simulink model "model_main4"  (R2024b)
settings: Solver=ode4  StartTime=0.0  StopTime=1000  FixedStep=dt  RelTol=1e-3
undefined symbols (not defined in the file): dt, Iws, m_tot, norm_Ib, Omega1_init, Omega2_init, Omega3_init, Omega4_init, qb0, rad2rpm, RCS_F, RCS_F_vec, RCS_Pos, RCS_pos, RCS_PWM_Freq, RCS_Sampling_time, RCS_THR_vec, REL_TS_POS_I_0, REL_TS_VEL_I_0, rpm2rad, RW_As, RW_Max_Speed, RW_t_max, SC_Ib, SC_state0, SS_Total_Mass, TC_Kepler, TS_Ib, TS_qb0, TS_state0, TS_wb0, wb0
libraries: simulink x16, simulink_extras x15, aerolibutil x8, sharedtransform x8
(part 2 of 3)

== matlab function model_main4/Subsystem/Attitude_PD_control1 ==
  settings: updateMethod=DISCRETE
  data: F_B_cmd output; r_I input; v_I input; q_IB input; r_d input; v_d input; a_d input; m input
function F_B_cmd  = CTRL_WRENCH_6DOF(r_I, v_I, q_IB, r_d, v_d, a_d, m)
%#codegen
% ============================================================
% Controller block
% Input :
%   r_I      [3x1] current position in inertial frame
%   v_I      [3x1] current velocity in inertial frame
%   q_IB     [4x1] quaternion [qw qx qy qz], Body -> Inertial
%   omega_B  [3x1] current angular velocity in body frame
%
%   r_d      [3x1] desired position in inertial frame
%   v_d      [3x1] desired velocity in inertial frame
%   a_d      [3x1] desired acceleration in inertial frame
%   q_d      [4x1] desired quaternion, Body -> Inertial
%   omega_d_B[3x1] desired angular velocity in body frame
%
%   m        scalar mass
%   J        [3x3] inertia matrix in body frame
%
% Output:
%   F_B_cmd    [3x1] desired total body force
%   tau_B_cmd  [3x1] desired total body torque
% ============================================================

    % -------------------------
    % Quaternion normalize
    % -------------------------
    q_IB = quat_normalize(q_IB); 

    % -------------------------
    % Gains (example)
    % -------------------------
    Kp_r = 10*diag([0.01, 0.006, 0.006]);   % position gain
    Kd_r = 100*diag([0.01, 0.01, 0.01]);   % velocity damping
 
    % Kp_r = diag([0.010, 0.010, 0.010]);   % position gain
    % Kd_r = diag([0.060, 0.060, 0.060]);   % velocity damping

    % -------------------------
    % Position control
    % inertial acceleration command
    % -------------------------
    e_r = r_I - r_d;
    e_v = v_I - v_d;

    a_cmd   = a_d - Kp_r * e_r - Kd_r * e_v;
    F_I_cmd = m * a_cmd;

    % Convert inertial force -> body force
    R_IB    = quat_to_rotm(q_IB);
    F_B_cmd = R_IB.' * F_I_cmd;
 
end


% ============================================================
% Local helper functions
% ============================================================

function qn = quat_normalize(q)
    n = norm(q);
    if n < 1e-12
        qn = [1;0;0;0];
    else
        qn = q / n;
    end
end
 

function R = quat_to_rotm(q)
    % q = [qw qx qy qz], Body -> Inertial
    qw = q(1); qx = q(2); qy = q(3); qz = q(4);

    R = [1-2*(qy^2+qz^2),   2*(qx*qy-qz*qw),   2*(qx*qz+qy*qw);
         2*(qx*qy+qz*qw),   1-2*(qx^2+qz^2),   2*(qy*qz-qx*qw);
         2*(qx*qz-qy*qw),   2*(qy*qz+qx*qw),   1-2*(qx^2+qy^2)];
end

== matlab function model_main4/Subsystem/Thruster Allocation ==
  settings: updateMethod=DISCRETE
  data: u_pwm output; F_B_cmd input; tau_B_cmd input; F_B_real output; tau_B_real output; r input; d input; F_max input
function [u_pwm, F_B_real, tau_B_real] = ALLOC_THRUSTER_PWM_16(F_B_cmd, tau_B_cmd, r, d, F_max)
%#codegen
% ============================================================
% Allocation block
% Input :
%   F_B_cmd    [3x1] desired total body force
%   tau_B_cmd  [3x1] desired total body torque
%
% Output:
%   u_pwm      [12x1] thruster duty command, 0 ~ 1
%   F_B_real   [3x1] realized body force after allocation
%   tau_B_real [3x1] realized body torque after allocation
%
% Example:
%   12-thruster layout for 6DoF control
%   Replace thruster geometry / Tmax below with your real spacecraft values.
% ============================================================

    % Build 6x12 thruster mapping matrix A
    A = build_thruster_matrix( 16, r, d, F_max);

    % Desired wrench
    w_cmd = [F_B_cmd; tau_B_cmd];

    % Bounded least-squares allocation: 0 <= u <= 1
    u_pwm = bounded_allocator_0_1(A, w_cmd);

    % Realized wrench
    w_real     = A * u_pwm;
    F_B_real   = w_real(1:3);
    tau_B_real = w_real(4:6);
end


% ============================================================
% Thruster layout
% ============================================================
function A = build_thruster_matrix(N, r, d, F_max)
    % --------------------------------------------------------
    % Example spacecraft half-size [m]
    % Replace with your real geometry
    % --------------------------------------------------------
    % L = 0.50;   % lever arm

    % --------------------------------------------------------
    % Max thrust of each thruster [N]
    % Replace with your real thruster max force
    % --------------------------------------------------------
    Tmax = F_max * ones(N,1);

    % --------------------------------------------------------
    % Thruster positions r_i in body frame [m]
    % Each column is one thruster position
    % --------------------------------------------------------
    % r = [ ...
    %      0,   0,   0,   0,   L,  -L,   L,  -L,   L,  -L,   L,  -L;
    %      L,  -L,   L,  -L,   0,   0,   0,   0,   L,   L,  -L,  -L;
    %      L,  -L,  -L,   L,   L,  -L,  -L,   L,   0,   0,   0,   0 ];

    % --------------------------------------------------------
    % Thruster unit directions d_i in body frame
    %
    % T1,T2 : +X
    % T3,T4 : -X
    % T5,T6 : +Y
    % T7,T8 : -Y
    % T9,T10: +Z
    % T11,T12:-Z
    % --------------------------------------------------------
    % d = [ ...
    %      1,   1,  -1,  -1,   0,   0,   0,   0,   0,   0,   0,   0;
    %      0,   0,   0,   0,   1,   1,  -1,  -1,   0,   0,   0,   0;
    %      0,   0,   0,   0,   0,   0,   0,   0,   1,   1,  -1,  -1 ];

    % --------------------------------------------------------
    % Build A = [F; tau], size 6x12
    % --------------------------------------------------------
    A = zeros(6,N);

    for i = 1:N
        f_i       = Tmax(i) * d(:,i);
        tau_i     = cross(r(:,i), f_i);
        A(:,i)    = [f_i; tau_i];
    end
end


% ============================================================
% Bounded allocator: 0 <= u <= 1
% Codegen-friendly fixed-size active-set style
% ============================================================
function u = bounded_allocator_0_1(A, w_cmd)
    N = 16;
    u = zeros(N,1);

    % free_mask(i)=true means this thruster is still free to solve
    free_mask = true(N,1);

    lambda = 1e-8;   % small damping

    for iter = 1:(N+1)

        % Residual after fixed/saturated thrusters
        w_res = w_cmd;
        for i = 1:N
            if ~free_mask(i)
                w_res = w_res - A(:,i) * u(i);
            end
        end

        % Collect free columns into Af (fixed-size construction)
        Af  = zeros(6,N);
        idx = zeros(N,1);
        nf  = 0;

        for i = 1:N
            if free_mask(i)
                nf = nf + 1;
                idx(nf) = i;
                Af(:,nf) = A(:,i);
            end
        end

        if nf == 0
            break;
        end

        % Minimum-norm damped solution on free set
        M       = Af * Af.' + lambda * eye(6);
        uf_full = Af.' * (M \ w_res);   % size Nx1, only first nf entries used

        % Put candidate solution into u
        for k = 1:nf
            i = idx(k);
            u(i) = uf_full(k);
        end

        % Check bounds and fix saturated variables
        violated = false;
        for k = 1:nf
            i = idx(k);

            if u(i) < 0
                u(i) = 0;
                free_mask(i) = false;
                violated = true;

            elseif u(i) > 1
                u(i) = 1;
                free_mask(i) = false;
                violated = true;
            end
        end

        if ~violated
            break;
        end
    end

    % Final clipping
    for i = 1:N
        if u(i) < 0
            u(i) = 0;
        elseif u(i) > 1
            u(i) = 1;
        end
    end
end

== matlab function model_main4/saturation ==
  data: max_speed input; res output; Omega_mea input; torque_cmd input
function res  = saturation(max_speed, Omega_mea, torque_cmd)

Omega1_mea = Omega_mea(1);
Omega2_mea = Omega_mea(2);
Omega3_mea = Omega_mea(3);
Omega4_mea = Omega_mea(4);

if abs(Omega1_mea)> max_speed
    res1 = 0;
else
    res1 = torque_cmd(1);
end

if abs(Omega2_mea)>max_speed
    res2 = 0;
else
    res2 = torque_cmd(2);
end

if abs(Omega3_mea)>max_speed
    res3 = 0;
else
    res3 = torque_cmd(3);
end

if abs(Omega4_mea)>max_speed
    res4 = 0;
else
    res4 = torque_cmd(4);
end

res = [res1,res2,res3,res4]';

end

== matlab function model_main4/TS 6-DOF Dynamics ==
  data: w input; x input; Ib input; wd output; T_ext input; F_ext input; xd output
function [wd, xd]  = eq_propagate(w, x, Ib, T_ext, F_ext)
% % 
% 출력 1: 위성 동체 좌표계 각가속도
% 출력 2: 관성좌표계 선가속도

%% Rotational Motion
% wd = [0 0 0]';
wd = inv(Ib)*(T_ext - cross(w, Ib*w));

%% Translational Motion


u  = 3.9860064e+14; % earth gravitional parameter
Re = 6378137;      % earth radius [m]

xd = zeros(size(x));

v1_i = x(4); % x1 = dx/dt
v2_i = x(5); % y1 = dy/dt
v3_i = x(6); % z1 = dz/dt
p1_i = x(1); % x
p2_i = x(2); % y
p3_i = x(3); % z

r=sqrt(p1_i^2+p2_i^2+p3_i^2);

% % %   Keplar Motion Equatnion
% % %  => r_dd + u/(r^3)r_ = 0 => r_dd = -u/(r^3)r_
xd(1) = v1_i;
xd(2) = v2_i;
xd(3) = v3_i;
xd(4) = -u*p1_i/(r^3) +  F_ext(1);
xd(5) = -u*p2_i/(r^3) +  F_ext(2);
xd(6) = -u*p3_i/(r^3) +  F_ext(3);

end

== matlab function model_main4/Subsystem/Attitude_PD_control2 ==
  settings: updateMethod=DISCRETE
  data: q_err input; omega_B input; omega_d_B input; J input; tau_B_cmd output
function tau_B_cmd  = CTRL_WRENCH_6DOF(q_err, omega_B, omega_d_B, J)
%#codegen
% ============================================================
% Controller block
% Input :
%   r_I      [3x1] current position in inertial frame
%   v_I      [3x1] current velocity in inertial frame
%   q_IB     [4x1] quaternion [qw qx qy qz], Body -> Inertial
%   omega_B  [3x1] current angular velocity in body frame
%
%   r_d      [3x1] desired position in inertial frame
%   v_d      [3x1] desired velocity in inertial frame
%   a_d      [3x1] desired acceleration in inertial frame
%   q_d      [4x1] desired quaternion, Body -> Inertial
%   omega_d_B[3x1] desired angular velocity in body frame
%
%   m        scalar mass
%   J        [3x3] inertia matrix in body frame
%
% Output:
%   F_B_cmd    [3x1] desired total body force
%   tau_B_cmd  [3x1] desired total body torque
% ============================================================
 
    % -------------------------
    % Gains (example)
    % -------------------------
    Kq   = J*diag([0.3, 0.3, 0.3]);   % attitude gain
    Kw   = J*diag([5, 5, 5]);   % angular-rate damping

    % Kq   = diag([10.0, 10.0, 10.0]);   % attitude gain
    % Kw   = diag([6.0,  6.0,  6.0 ]);   % angular-rate damping
    % -------------------------
 
    % -------------------------
    % Attitude control 
    % -------------------------
 
    % shortest-path quaternion
    if q_err(1) < 0
        q_err = -q_err;
    end

    e_w = omega_B - omega_d_B;

    % PD + gyro compensation
    tau_B_cmd = -Kq * q_err(2:4) ...
                -Kw * e_w ...
                +cross(omega_B, J * omega_B);
end


% ============================================================
% Local helper functions
% ============================================================

function qn = quat_normalize(q)
    n = norm(q);
    if n < 1e-12
        qn = [1;0;0;0];
    else
        qn = q / n;
    end
end

function qc = quat_conj(q)
    qc = [q(1); -q(2); -q(3); -q(4)];
end

function q = quat_mul(q1, q2)
    % Hamilton product
    w1 = q1(1); x1 = q1(2); y1 = q1(3); z1 = q1(4);
    w2 = q2(1); x2 = q2(2); y2 = q2(3); z2 = q2(4);

    q = [ w1*w2 - x1*x2 - y1*y2 - z1*z2;
          w1*x2 + x1*w2 + y1*z2 - z1*y2;
          w1*y2 - x1*z2 + y1*w2 + z1*x2;
          w1*z2 + x1*y2 - y1*x2 + z1*w2 ];
end

== matlab function model_main4/RCS_Position&Attitude_Controller ==
  settings: updateMethod=DISCRETE
  data: r_rel input; v_rel input; r_ref input; v_ref input; a_ref input; q input; q_err input; w_err input; wb input; F_cmd_B output; tau_cmd_B output; m_sc input; Ib input; Kp_pos input; Kd_pos input; Kp_att input; Kd_att input; r_err output; v_err output; q output; q_err_vec output; w_err output; a_cmd output
function [F_cmd_B, tau_cmd_B, r_err, v_err, q, q_err_vec, w_err, a_cmd] = ...
    relative_position_los_controller( ...
    r_rel, v_rel, ...          % [3x1] relative position/velocity
    r_ref, v_ref, a_ref, ...   % [3x1] desired relative pos/vel/acc
    q, q_err, w_err, wb, m_sc, Ib, Kp_pos, Kd_pos, Kp_att, Kd_att)
%#codegen
%
% q, q_los_ref : scalar-first quaternion [qw qx qy qz]'
%                body -> reference
% r_rel, r_ref, v_rel, v_ref, a_ref : reference frame 기준
%
% 출력:
% F_cmd_B   : [3x1] body frame force command
% tau_cmd_B : [3x1] body frame torque command

F_cmd_B   = zeros(3,1);
tau_cmd_B = zeros(3,1);
r_err     = zeros(3,1);
v_err     = zeros(3,1);
q_err_vec = zeros(3,1);
% w_err     = zeros(3,1);
a_cmd     = zeros(3,1);

%% 1) Relative position controller
r_err = r_ref - r_rel;
v_err = v_ref - v_rel;

a_cmd = a_ref + Kp_pos * r_err + Kd_pos * v_err;
F_cmd_R = m_sc * a_cmd;

%% 2) Reference frame -> body frame
% q : body -> reference
% therefore F_B = C_BR' * F_R
C_BR   = quat_to_dcm_sf(q);
F_cmd_B = C_BR' * F_cmd_R;

%% 3) LOS attitude controller

% shortest path
% if q_err(1) < 0
%     q_err = -q_err;
% end

q_err_vec = q_err(2:4);

tau_cmd_B = Kp_att * q_err_vec + Kd_att * w_err + cross(wb, Ib*wb);
end


function q_out = quat_mul_sf(a, b)
% scalar-first quaternion multiplication
q_out = [ a(1)*b(1) - a(2)*b(2) - a(3)*b(3) - a(4)*b(4);
    a(1)*b(2) + a(2)*b(1) + a(3)*b(4) - a(4)*b(3);
    a(1)*b(3) - a(2)*b(4) + a(3)*b(1) + a(4)*b(2);
    a(1)*b(4) + a(2)*b(3) - a(3)*b(2) + a(4)*b(1) ];
end


function C = quat_to_dcm_sf(q)
% scalar-first quaternion, body -> reference
q = q / (sqrt(sum(q.^2)) + 1e-12);

qw = q(1);
qx = q(2);
qy = q(3);
qz = q(4);

C = [1-2*(qy*qy+qz*qz),   2*(qx*qy-qw*qz),   2*(qx*qz+qw*qy);
    2*(qx*qy+qw*qz),     1-2*(qx*qx+qz*qz), 2*(qy*qz-qw*qx);
    2*(qx*qz-qw*qy),     2*(qy*qz+qw*qx),   1-2*(qx*qx+qy*qy)];
end

== matlab function model_main4/RCS_Force_Torque_Allocation ==
  settings: updateMethod=DISCRETE
  data: F_cmd input; tau_cmd input; RCS_pos input; RCS_F_vec input; Tmax input; duty output; F_est output; tau_est output; F_err output; tau_err output; sat_ratio output; wF input; wT input
function [duty, F_est, tau_est, F_err, tau_err, sat_ratio] = ...
    rcs_force_torque_allocator(F_cmd, tau_cmd, RCS_pos, RCS_F_vec, Tmax, wF, wT)
%#codegen
%
% F_cmd      : [3x1] commanded force in body frame [N]
% tau_cmd    : [3x1] commanded torque in body frame [N*m]
% RCS_pos    : [3xN] thruster positions in body frame [m]
% RCS_F_vec  : [3xN] thruster direction vectors
% Tmax       : scalar, max thrust of one thruster [N]
% wF         : scalar, force tracking weight
% wT         : scalar, torque tracking weight
%
% duty       : [N x 1], 0~1
% F_est      : [3x1], achieved force [N]
% tau_est    : [3x1], achieved torque [N*m]
% F_err      : [3x1], force error [N]
% tau_err    : [3x1], torque error [N*m]
% sat_ratio  : saturated thruster ratio

    N = size(RCS_pos, 2);

    duty      = zeros(N,1);
    F_est     = zeros(3,1);
    tau_est   = zeros(3,1);
    F_err     = zeros(3,1);
    tau_err   = zeros(3,1);
    sat_ratio = 0;

    Fmat = zeros(3, N);
    Tmat = zeros(3, N);

    for i = 1:N
        dir_i = RCS_F_vec(:,i);
        nrm   = sqrt(sum(dir_i.^2));

        if nrm > 1e-12
            dir_i = dir_i / nrm;
        else
            dir_i = [0;0;0];
        end

        Fi = Tmax * dir_i;
        Ti = cross3(RCS_pos(:,i), Fi);

        Fmat(:,i) = Fi;
        Tmat(:,i) = Ti;
    end

    % Solve:
    % min || wF*(Fmat*u - F_cmd) ||^2 + || wT*(Tmat*u - tau_cmd) ||^2
    % s.t. 0 <= u <= 1

    A = [wF * Fmat;
         wT * Tmat];

    b = [wF * F_cmd;
         wT * tau_cmd];

    H = A' * A + 1e-8 * eye(N);
    g = A' * b;

    alpha = 1.0 / (trace(H) + 1e-9);
    u = zeros(N,1);

    for k = 1:150
        grad = H * u - g;
        u    = u - alpha * grad;

        for j = 1:N
            if u(j) < 0
                u(j) = 0;
            elseif u(j) > 1
                u(j) = 1;
            end
        end
    end

    duty    = u;
    F_est   = Fmat * duty;
    tau_est = Tmat * duty;

    F_err   = F_cmd   - F_est;
    tau_err = tau_cmd - tau_est;

    sat_ratio = sum(duty > 0.999) / N;
end


function c = cross3(a, b)
    c = [ a(2)*b(3) - a(3)*b(2);
          a(3)*b(1) - a(1)*b(3);
          a(1)*b(2) - a(2)*b(1) ];
end

== matlab function model_main4/Mission_Supporter ==
  settings: updateMethod=DISCRETE
  data: flag output; res_pos input; stop output; Los_angle input
function [flag, stop]  = Mission_Supporter(res_pos, Los_angle)
persistent prev_flag

if isempty(prev_flag)
    prev_flag = 0;
end

d_norm = norm(res_pos);
d_parking = 5;


if d_norm - d_parking > 1 
    prev_flag = 0; % approach, RCS on
else
    if prev_flag == 0 && Los_angle < 0.2
        prev_flag = 1; % station keeping, RW on
    end
end
 
flag= prev_flag;
 

% 종료 조건
if d_norm <= 0.1
    stop = 1;
else
    stop = 0;
end

== matlab function model_main4/command_generator ==
  settings: updateMethod=DISCRETE
  data: rel_p_cmd output; flag input; rel_v_cmd output; Kp_pos output; Kd_pos output
function [rel_p_cmd,rel_v_cmd,Kp_pos,Kd_pos]  = Mission_Supporter(flag)

if flag == 0
    rel_p_cmd = [5 0 0]';
    rel_v_cmd = [0 0 0]';
    Kp_pos = 0.3;
    Kd_pos = 18.0;
else
    rel_p_cmd = [1 0 0]';
    rel_v_cmd = [0 0 0]';
    Kp_pos = 0.3;
    Kd_pos = 18.0;    
end


end

== matlab function model_main4/Get LOS Quaternion ==
  data: r_rel input; q output; ang_deg output; axis_rot output
function [q, ang_deg, axis_rot] = boresight_to_target_quat(r_rel)
%#codegen
% ============================================================
% boresight_to_target_quat
%
% Input:
%   r_rel    [3x1] : relative position vector
%
% Output:
%   q        [4x1] : quaternion [w; x; y; z]
%                    rotating boresight [1;0;0] to r_rel direction
%   ang_deg  [1x1] : rotation angle in degrees
%   axis_rot [3x1] : rotation axis (unit vector)
%
% Notes:
%   - boresight reference is fixed as [1; 0; 0]
%   - quaternion is scalar-first
%   - handles parallel / anti-parallel edge cases
% ============================================================

    % Reference boresight
    b_ref = [1; 0; 0];

    % Small threshold
    eps_val = 1e-12;

    % Check input norm
    r_norm = norm(r_rel);
    if r_norm < eps_val
        % Undefined direction
        q = [1; 0; 0; 0];
        ang_deg = 0;
        axis_rot = [1; 0; 0];
        return;
    end

    % Normalize target direction
    v = r_rel / r_norm;
    u = b_ref;

    % Dot product
    c = dot(u, v);
    c = max(min(c, 1.0), -1.0);   % numerical safety

    % Case 1: same direction
    if c > 1 - 1e-10
        q = [1; 0; 0; 0];
        ang_deg = 0;
        axis_rot = [1; 0; 0];
        return;
    end

    % Case 2: opposite direction
    if c < -1 + 1e-10
        % Need 180 deg rotation about any axis orthogonal to [1;0;0]
        % Choose y-axis
        axis_rot = [0; 1; 0];
        q = [0; axis_rot];   % cos(pi/2)=0, sin(pi/2)=1
        ang_deg = 180;
        return;
    end

    % General case
    cross_uv = cross(u, v);

    % Robust quaternion from two vectors:
    % q = [1 + dot(u,v); cross(u,v)] then normalize
    q = [1 + c;
         cross_uv(1);
         cross_uv(2);
         cross_uv(3)];

    q = q / norm(q);

    % Rotation angle
    ang_rad = 2 * acos(q(1));
    ang_deg = ang_rad * 180 / pi;

    % Rotation axis
    s = sqrt(1 - q(1)^2);
    if s < 1e-10
        axis_rot = [1; 0; 0];
    else
        axis_rot = q(2:4) / s;
    end
end

== matlab function model_main4/Enabled Subsystem/QP Controller ==
  settings: updateMethod=DISCRETE
  data: tau_pd input; u_rw_cmd output; Omega_rw input; RW_max_speed input; tau_rcs_max input; eta_rcs input; v1 input; v2 input; dt input; tau_rcs_cmd output; tau_rw_body output; tau_dump_ref output; s1 output; s2 output; exitflag_out output
function [u_rw_cmd, tau_rcs_cmd, tau_rw_body, tau_dump_ref, s1, s2, exitflag_out] = ...
    QP_Controller(tau_pd, Omega_rw, RW_max_speed, tau_rcs_max, eta_rcs, v1, v2, dt)
 
% QP with two slack variables:
%   s1 : attitude torque slack
%   s2 : dumping torque slack
%
% Inputs
%   tau_pd       [3x1] desired total body torque from PD [N*m]
%   Omega_rw     [4x1] current wheel speeds [rad/s]
%   RW_max_speed [1x1] wheel speed limit [rad/s]
%   tau_rcs_max  [3x1] approximate RCS body torque bound [N*m]
%   eta_rcs      [1x1] RCS effort weight
%   v1           [1x1] attitude slack weight
%   v2           [1x1] dumping slack weight
%   dt           [1x1] sample time [s]
%
% Outputs
%   u_rw_cmd     [4x1] RW wheel torque command [N*m]
%   tau_rcs_cmd  [3x1] RCS dumping body torque command [N*m]
%   tau_rw_body  [3x1] RW body torque [N*m]
%   tau_dump_ref [3x1] desired dumping torque reference [N*m]
%   s1           [3x1] attitude torque slack [N*m]
%   s2           [3x1] dumping torque slack [N*m]
%   exitflag_out [1x1] quadprog exitflag

persistent u_save;

if isempty(u_save)
    u_save = zeros(13,1);
end
 
u_prev   = u_save;

tau_pd      = reshape(tau_pd,      [3,1]);
Omega_rw    = reshape(Omega_rw,    [4,1]);
tau_rcs_max = reshape(tau_rcs_max, [3,1]);
Omega_ref = 1000 * pi/30 * ones(4,1);

%% RW geometry from current model
% tau_rw_body = -As * u_rw_cmd
As = [ 0.70710678,  0.0,        -0.70710678,  0.0;
       0.0,         0.70710678,  0.0,        -0.70710678;
       0.70710678,  0.70710678,  0.70710678,  0.70710678 ];

Iws = 0.227 * eye(4);

%% wheel limits
% Wheel torque limits [N*m]
u_rw_max = 0.5 * ones(4,1);
u_rw_min = -u_rw_max;

% Wheel torque rate limits [N*m/s]
du_max = [0.50; 0.50; 0.50; 0.50]*100;
du_min = -du_max;

% Wheel speed limits [rad/s]
Omega_max = RW_max_speed * ones(4,1);
Omega_min = -Omega_max;

%% dumping reference
% % saturation ratio
% sat_ratio = max(abs(Omega_rw) ./ (Omega_max + 1e-12));
% 
% % activation factor alpha
% if sat_ratio <= sat_start
%     alpha = 0.0;
% else
%     alpha = (sat_ratio - sat_start) / (1.0 - sat_start);
%     if alpha > 1.0
%         alpha = 1.0;
%     end
% end
alpha =  0;
tau_dump_ref = -alpha * As * Iws * (Omega_rw - Omega_ref);

% % approximate RCS torque clipping
% for i = 1:3
%     if tau_dump_ref(i) > tau_rcs_max(i)
%         tau_dump_ref(i) = tau_rcs_max(i);
%     elseif tau_dump_ref(i) < -tau_rcs_max(i)
%         tau_dump_ref(i) = -tau_rcs_max(i);
%     end
% end

%% decision variable
% z = [u_rw(4); tau_rcs(3); s1(3); s2(3)]  => total 13

%% cost

Wu   = eye(4);
Wrcs = eta_rcs * eye(3);
V1   = v1      * eye(3);
V2   = v2      * eye(3);

H = blkdiag(Wu, Wrcs, V1, V2);
H = 0.5*(H + H') + 1e-9*eye(13);

f = zeros(13,1);

%% equality constraints
% 1) attitude torque:
%    -As*u_rw + tau_rcs - s1 = tau_pd
%
% 2) dumping torque:
%    tau_rcs - s2 = tau_dump_ref

Aeq = [       -As, eye(3),     -eye(3), zeros(3,3);
       zeros(3,4), eye(3),  zeros(3,3),    -eye(3)];

beq = [      tau_pd;
       tau_dump_ref];

%% bounds
% RW torque bounds
% Torque-rate bounds
lb_rate = u_prev(1:4) + du_min * dt;
ub_rate = u_prev(1:4) + du_max * dt;

% Speed-next bounds
% Omega_next = Omega_rw + dt*(u./Jw)
% => u >= Jw .* (Omega_min - Omega_rw)/dt
% => u <= Jw .* (Omega_max - Omega_rw)/dt
lb_speed = diag(Iws) .* ((Omega_min - Omega_rw) / dt);
ub_speed = diag(Iws) .* ((Omega_max - Omega_rw) / dt);

% Final bounds
lb_u = inf*max(u_rw_min, max(lb_rate, lb_speed));
ub_u = min(u_rw_max, min(ub_rate, ub_speed));

% Feasibility repair
% for i = 1:4
%     if lb_u(i) > ub_u(i)
%         c = 0.5 * (lb_u(i) + ub_u(i));
%         lb_u(i) = c;
%         ub_u(i) = c;
%     end
% end


% RCS torque bounds
% lb_t = -tau_rcs_max;
% ub_t =  tau_rcs_max;
lb_t = -inf*ones(3,1);
ub_t =  inf*ones(3,1);

% slack bounds
big = 1e6;  % inf
lb_s1 = -big * ones(3,1);
ub_s1 =  big * ones(3,1);
lb_s2 = -big * ones(3,1);
ub_s2 =  big * ones(3,1);

lb = [lb_u; lb_t; lb_s1; lb_s2];
ub = [ub_u; ub_t; ub_s1; ub_s2];

%% initial guess
x0 = [zeros(4,1);
      zeros(3,1);
      -tau_pd;
      -tau_dump_ref];
% rw : Omegad cmd, rcs : tau cmd, 
% x0 = min(max(u_prev, lb), ub);

%% solve
options = optimoptions('quadprog', ...
    'Algorithm', 'active-set', ...
    'Display', 'off', ...
    'ConstraintTolerance', 1e-6, ...
    'OptimalityTolerance', 1e-6, ...
    'StepTolerance', 1e-12, ...
    'MaxIterations', 50);

[z, ~, exitflag] = quadprog(H, f, [], [], Aeq, beq, lb, ub, x0, options);

if isempty(z) || exitflag <= 0
    z = x0;
end

%% outputs
u_rw_cmd    = z(1:4);
tau_rcs_cmd = z(5:7);
s1          = z(8:10);
s2          = z(11:13);

tau_rw_body = -As * u_rw_cmd;
% tau_total   = tau_rw_body + tau_rcs_cmd;
u_save = z;
exitflag_out = exitflag;
end

== matlab function model_main4/Enabled Subsystem/QP Controller1 ==
  settings: updateMethod=DISCRETE
  data: tau_pd_in input; u_rw_cmd output; Omega_rw_in input; Omega_ref_in input; RW_max_speed input; tau_rcs_max_in input; k_dump input; eta_rw input; eta_rcs input; v1 input; v2 input; dt input; tau_rcs_cmd output; tau_rw_body output; tau_dump_ref output; s1 output; s2 output; exitflag_out output
function [u_rw_cmd, tau_rcs_cmd, tau_rw_body, tau_dump_ref, s1, s2, exitflag_out] = ...
    QP_CA_RW_RCS3(tau_pd_in, Omega_rw_in, Omega_ref_in, ...
                  RW_max_speed, tau_rcs_max_in, ...
                  k_dump, eta_rw, eta_rcs, v1, v2, dt)
%#codegen
%
% QP control allocation based on the structure of Sec. 3.1,
% simplified to:
%   - RW (internal actuator)
%   - lumped 3-axis external torque command (for later RCS allocation)
%
% Decision variable:
%   z = [u_rw(4); tau_rcs(3); s1(3); s2(3)]  -> 13 states
%
% Equality constraints:
%   -As*u_rw + tau_rcs - s1 = tau_pd
%    tau_rcs - s2           = tau_dump_ref
%
% Inputs
%   tau_pd_in      [3x1] desired attitude body torque from high-level controller [N*m]
%   Omega_rw_in    [4x1] current RW speeds [rad/s]
%   Omega_ref_in   [4x1] desired RW speed reference [rad/s]
%   RW_max_speed   [1x1] RW speed limit [rad/s]
%   tau_rcs_max_in [3x1] max body torque envelope available from RCS [N*m]
%   k_dump         [1x1] momentum dumping gain [1/s]
%   eta_rw         [1x1] RW effort weight
%   eta_rcs        [1x1] external torque effort weight
%   v1             [1x1] attitude slack weight
%   v2             [1x1] dumping slack weight
%   dt             [1x1] sample time [s]
%
% Outputs
%   u_rw_cmd       [4x1] RW motor torque command [N*m]
%   tau_rcs_cmd    [3x1] desired 3-axis body torque for RCS allocation [N*m]
%   tau_rw_body    [3x1] body torque generated by RW [N*m]
%   tau_dump_ref   [3x1] desired external dumping torque [N*m]
%   s1             [3x1] attitude torque slack
%   s2             [3x1] dumping torque slack
%   exitflag_out   [1x1] quadprog exitflag

persistent z_save;

if isempty(z_save)
    z_save = zeros(13,1);
end

%% outputs
u_rw_cmd     = zeros(4,1);
tau_rcs_cmd  = zeros(3,1);
tau_rw_body  = zeros(3,1);
tau_dump_ref = zeros(3,1);
s1           = zeros(3,1);
s2           = zeros(3,1);
exitflag_out = 0;

%% fixed-size local copies
tau_pd = zeros(3,1);
tau_pd(1) = tau_pd_in(1);
tau_pd(2) = tau_pd_in(2);
tau_pd(3) = tau_pd_in(3);

Omega_rw = zeros(4,1);
Omega_rw(1) = Omega_rw_in(1);
Omega_rw(2) = Omega_rw_in(2);
Omega_rw(3) = Omega_rw_in(3);
Omega_rw(4) = Omega_rw_in(4);

Omega_ref = zeros(4,1);
Omega_ref(1) = Omega_ref_in(1);
Omega_ref(2) = Omega_ref_in(2);
Omega_ref(3) = Omega_ref_in(3);
Omega_ref(4) = Omega_ref_in(4);

tau_rcs_max = zeros(3,1);
tau_rcs_max(1) = abs(tau_rcs_max_in(1));
tau_rcs_max(2) = abs(tau_rcs_max_in(2));
tau_rcs_max(3) = abs(tau_rcs_max_in(3));

if dt <= 1e-6
    dt = 1e-6;
end

if RW_max_speed <= 1e-6
    RW_max_speed = 1e-6;
end

%% RW geometry
% tau_rw_body = -As * u_rw
As = [ 0.70710678,  0.0,        -0.70710678,  0.0;
       0.0,         0.70710678,  0.0,        -0.70710678;
       0.70710678,  0.70710678,  0.70710678,  0.70710678 ];

% wheel spin inertias [kg*m^2]
Jw = 0.227 * ones(4,1);

%% actuator limits
% RW torque limits
u_rw_max = 0.2 * ones(4,1);
u_rw_min = -u_rw_max;

% RW torque-rate limits
du_max = 2.0 * ones(4,1);   % [N*m/s]
du_min = -du_max;

% RW speed limits
Omega_max = RW_max_speed * ones(4,1);
Omega_min = -Omega_max;

%% previous solution
z_prev = z_save;
u_prev = z_prev(1:4);

%% virtual momentum dumping torque
% Paper uses u_h = -k_h * (...) * Cw*Jw*omega_w,e
% Here simplified for RCS-only external torque:
%   tau_dump_ref = -k_dump * h_rw_err
% where h_rw_err = As * diag(Jw) * (Omega_rw - Omega_ref)

omega_err = Omega_rw - Omega_ref;
h_rw_err  = As * (Jw .* omega_err);   % [N*m*s]
tau_dump_ref = -k_dump * h_rw_err;    % [N*m]

%% QP cost
% z = [u_rw(4); tau_rcs(3); s1(3); s2(3)]
H = zeros(13,13);
f = zeros(13,1);

% effort weights
H(1,1) = 2*eta_rw; H(2,2) = 2*eta_rw; H(3,3) = 2*eta_rw; H(4,4) = 2*eta_rw;
H(5,5) = 2*eta_rcs; H(6,6) = 2*eta_rcs; H(7,7) = 2*eta_rcs;
H(8,8) = 2*v1; H(9,9) = 2*v1; H(10,10) = 2*v1;
H(11,11) = 2*v2; H(12,12) = 2*v2; H(13,13) = 2*v2;

% optional small RW smoothing
wr = 1e-3;
H(1,1) = H(1,1) + 2*wr;
H(2,2) = H(2,2) + 2*wr;
H(3,3) = H(3,3) + 2*wr;
H(4,4) = H(4,4) + 2*wr;

f(1:4) = -2*wr*u_prev;

% numerical symmetry
H = 0.5*(H + H') + 1e-9*eye(13);

%% equality constraints
% -As*u_rw + tau_rcs - s1 = tau_pd
%  tau_rcs - s2           = tau_dump_ref

Aeq = [      -As, eye(3),    -eye(3), zeros(3,3);
       zeros(3,4), eye(3), zeros(3,3),   -eye(3)];

beq = [tau_pd;
       tau_dump_ref];

%% bounds
% RW torque-rate bounds
lb_rate = u_prev + du_min * dt;
ub_rate = u_prev + du_max * dt;

% RW speed-next bounds
% Omega_next = Omega_rw + dt*(u_rw./Jw)
lb_speed = Jw .* ((Omega_min - Omega_rw) / dt);
ub_speed = Jw .* ((Omega_max - Omega_rw) / dt);

% final RW bounds
lb_u = max(u_rw_min, max(lb_rate, lb_speed));
ub_u = min(u_rw_max, min(ub_rate, ub_speed));

% feasibility repair
for i = 1:4
    if lb_u(i) > ub_u(i)
        c = 0.5 * (lb_u(i) + ub_u(i));
        lb_u(i) = c;
        ub_u(i) = c;
    end
end

% external torque bounds
lb_t = -tau_rcs_max;
ub_t =  tau_rcs_max;

% slack bounds
big = 1e6;
lb_s1 = -big * ones(3,1);
ub_s1 =  big * ones(3,1);
lb_s2 = -big * ones(3,1);
ub_s2 =  big * ones(3,1);

lb = [lb_u; lb_t; lb_s1; lb_s2];
ub = [ub_u; ub_t; ub_s1; ub_s2];

%% initial guess (make it equality-feasible)
u0 = min(max(u_prev, lb_u), ub_u);

t0 = tau_dump_ref;
for i = 1:3
    if t0(i) > ub_t(i)
        t0(i) = ub_t(i);
    elseif t0(i) < lb_t(i)
        t0(i) = lb_t(i);
    end
end

s10 = -As*u0 + t0 - tau_pd;
s20 = t0 - tau_dump_ref;

x0 = [u0;
      t0;
      s10;
      s20];

%% solve
A = zeros(0,13);
b = zeros(0,1);

options = optimoptions('quadprog', ...
    'Algorithm', 'active-set', ...
    'Display', 'off', ...
    'ConstraintTolerance', 1e-6, ...
    'OptimalityTolerance', 1e-6, ...
    'StepTolerance', 1e-12, ...
    'MaxIterations', 50);

[z, ~, exitflag] = quadprog(H, f, A, b, Aeq, beq, lb, ub, x0, options);

if isempty(z) || exitflag <= 0
    z = x0;
end

%% outputs
u_rw_cmd    = z(1:4);
tau_rcs_cmd = z(5:7);
s1          = z(8:10);
s2          = z(11:13);

tau_rw_body = -As * u_rw_cmd;

z_save = z;
exitflag_out = exitflag;

end

== matlab function model_main4/Subsystem/Attitude_PD_control ==
  settings: updateMethod=DISCRETE
  data: u_torq output; q_err input; w_err input
function u_torq = att_pd_control(q_err, w_err)

persistent first_flg
persistent I_save

dt = 0.01;

if isempty(first_flg)
    first_flg = 1;
    I_save = [0 0 0]';
end

K1 = 10.1*diag([1 1 1]);
K2 = 8.2*diag([1 1 1]);
K3 = 0.1*diag([1 1 1]);

q_err_ = [q_err(2), q_err(3), q_err(4)]';

u_torq = K1*q_err_ + K2*w_err + K3*I_save;

I_save = I_save + q_err_ * dt;

end

== matlab function model_main4/Subsystem/THR_Allocation ==
  data: pwm output; tau_cmd input; F_on input; f input; r_thr input
function pwm = RCS_Torque2PWM(tau_cmd, F_on, f, r_thr)
%#codegen
% ============================================================
% Minimal RCS allocation: torque command -> PWM duty (0..1)
%   tau ≈ sum_i r_i x (f_i * F_on_i * pwm_i)
%
% Inputs:
%   tau_cmd [3x1]
%   F_on    scalar or [12x1]
%   f       [3x12]  (columns are unit vectors)
%   r_thr   [3x12]  (columns are position vectors wrt CoM)
%
% Output:
%   pwm     [12x1] duty in [0,1]
% ============================================================
N = 16;
% F_on -> 12x1
if isscalar(F_on)
    Fon = F_on * ones(N,1);
else
    Fon = F_on(:);
end

% Build effectiveness matrix B (3x12): tau = B * pwm
B = zeros(3,N);
for i = 1:N
    Fi = Fon(i);
    B(:,i) = cross3(r_thr(:,i), f(:,i) * Fi);  % torque from pwm=1
end

% Unconstrained least-squares solution (minimum-norm)
pwm = B' * ((B*B') \ tau_cmd);

% Clamp to [0,1]
for i=1:N
    if pwm(i) < 0, pwm(i) = 0; end
    if pwm(i) > 1, pwm(i) = 1; end
end

end

function c = cross3(a,b)
c = [ a(2)*b(3) - a(3)*b(2);
      a(3)*b(1) - a(1)*b(3);
      a(1)*b(2) - a(2)*b(1) ];
end

== matlab function model_main4/Quaternion_Kinematics ==
  data: w input; qd output; q input
function qd = fcn(w,q)

F_q = (1/2)*[0 -w(1) -w(2) -w(3);
       w(1) 0 w(3) -w(2);
       w(2) -w(3) 0 w(1);
       w(3) w(2) -w(1) 0];

qd = F_q*q;

end

== matlab function model_main4/Enabled Subsystem/QP  ==
  settings: updateMethod=DISCRETE
  data: tau_des input; u_rw_cmd output; Omega_rw input; dt input; tau_body_cmd output; exitflag_out output; RW_max_speed input; Iws input; As input
function [u_rw_cmd, tau_body_cmd, exitflag_out] = RW4_QP_Controller(tau_des, Omega_rw, dt, RW_max_speed, Iws, As)
%#codegen
%
% 4-wheel Reaction Wheel QP controller
% tau_body = -A_rw * u_rw
%
% Inputs:
%   tau_des   [3x1] desired body torque
%   Omega_rw  [4x1] current wheel speeds [rad/s]
%   u_prev    [4x1] previous wheel torque command [N*m]
%   dt        scalar control period [s]
%
% Outputs:
%   u_rw_cmd     [4x1] wheel motor torque command
%   tau_body_cmd [3x1] actual body torque from RW
%   exitflag_out scalar

persistent u_save;

if isempty(u_save)
    u_save = [0 0 0 0]';
end

u_rw_cmd     = zeros(4,1);
tau_body_cmd = zeros(3,1);
exitflag_out = 0;

tau_des  = reshape(tau_des,  [3,1]);
Omega_rw = reshape(Omega_rw, [4,1]);
u_prev   = u_save;

% =========================
% RW axis matrix (3x4)
% =========================
A_rw = [ 0.70710678,  0.0,        -0.70710678,  0.0;
         0.0,         0.70710678,  0.0,        -0.70710678;
         0.70710678,  0.70710678,  0.70710678,  0.70710678 ];

% =========================
% User parameters
% =========================
% Torque tracking weight (body torque tracking)
Wtau = diag([10.0, 10.0, 10.0]);

% Wheel torque magnitude penalty
Wu = 1e-3 * eye(4);

% Wheel torque smoothing penalty
Wr = 1e-2 * eye(4);

% Optional wheel-speed centering penalty
% Start with very small values. Increase later if wheel speeds drift too much.
Wh = zeros(4,4);
% 예: Wh = 1e-6 * eye(4);

% Wheel inertia about spin axis [kg*m^2]
Jw = 0.227*[1;1;1;1];

% Wheel torque limits [N*m]
u_max = [0.2; 0.2; 0.2; 0.2];
u_min = -u_max;

% Wheel torque rate limits [N*m/s]
du_max = [0.20; 0.20; 0.20; 0.20];
du_min = -du_max;

% Wheel speed limits [rad/s]
Omega_max = [RW_max_speed;RW_max_speed;RW_max_speed;RW_max_speed];
Omega_min = -Omega_max;

% =========================
% QP construction
%
% minimize 0.5*|| -A_rw*u - tau_des ||^2_Wtau
%        + 0.5*u'*Wu*u
%        + 0.5*(u-u_prev)'*Wr*(u-u_prev)
%        + 0.5*(Omega_next)'*Wh*(Omega_next)
%
% Omega_next = Omega_rw + D*u
% D = diag(dt./Jw)
% =========================

D = diag(dt ./ Jw);

H = A_rw' * Wtau * A_rw + Wu + Wr + D' * Wh * D;
f = A_rw' * Wtau * tau_des - Wr * u_prev + D' * Wh * Omega_rw;

% Make H numerically symmetric
H = 0.5 * (H + H');

% =========================
% Constraints
% 1) wheel torque bounds
% 2) wheel torque rate bounds
% 3) next-step wheel speed bounds
% =========================

% Torque-rate bounds
lb_rate = u_prev + du_min * dt;
ub_rate = u_prev + du_max * dt;

% Speed-next bounds
% Omega_next = Omega_rw + dt*(u./Jw)
% => u >= Jw .* (Omega_min - Omega_rw)/dt
% => u <= Jw .* (Omega_max - Omega_rw)/dt
lb_speed = Jw .* ((Omega_min - Omega_rw) / dt);
ub_speed = Jw .* ((Omega_max - Omega_rw) / dt);

% Final bounds
lb = max(u_min, max(lb_rate, lb_speed));
ub = min(u_max, min(ub_rate, ub_speed));

% Feasibility repair
for i = 1:4
    if lb(i) > ub(i)
        c = 0.5 * (lb(i) + ub(i));
        lb(i) = c;
        ub(i) = c;
    end
end

% Empty linear inequality/equality constraints
A   = zeros(0,4);
b   = zeros(0,1);
Aeq = zeros(0,4);
beq = zeros(0,1);

% Initial guess for active-set
x0 = min(max(u_prev, lb), ub);

% quadprog codegen-friendly option
options = optimoptions('quadprog', ...
    'Algorithm', 'active-set', ...
    'ConstraintTolerance', 1e-6, ...
    'OptimalityTolerance', 1e-6, ...
    'StepTolerance', 1e-12, ...
    'MaxIterations', 50);

[u_sol, ~, exitflag] = quadprog(H, f, A, b, Aeq, beq, lb, ub, x0, options);

if exitflag <= 0 || isempty(u_sol)
    u_rw_cmd = x0;
else
    u_rw_cmd = u_sol;
end

tau_body_cmd = -A_rw * u_rw_cmd;
u_save = u_rw_cmd;
exitflag_out = exitflag;

== matlab function model_main4/Subsystem/Get LOS Quaternion7 ==
  settings: updateMethod=DISCRETE
  data: r_rel input; v_rel input; r_ref input; v_ref input; a_ref input; q input; q_err input; w_err input; F_cmd_B output; tau_cmd_B output; m_sc input; Kp_pos input; Kd_pos input; Kp_att input; Kd_att input; r_err output; v_err output; q output; q_err_vec output; w_err output; a_cmd output
function [F_cmd_B, tau_cmd_B, r_err, v_err, q, q_err_vec, w_err, a_cmd] = ...
    relative_position_los_controller( ...
    r_rel, v_rel, ...          % [3x1] relative position/velocity
    r_ref, v_ref, a_ref, ...   % [3x1] desired relative pos/vel/acc
    q, q_err, w_err, ...                  % [4x1], [3x1] current attitude/angular velocity
    m_sc, Kp_pos, Kd_pos, Kp_att, Kd_att)
%#codegen
%
% q, q_los_ref : scalar-first quaternion [qw qx qy qz]'
%                body -> reference
% r_rel, r_ref, v_rel, v_ref, a_ref : reference frame 기준
%
% 출력:
% F_cmd_B   : [3x1] body frame force command
% tau_cmd_B : [3x1] body frame torque command

    F_cmd_B   = zeros(3,1);
    tau_cmd_B = zeros(3,1);
    r_err     = zeros(3,1);
    v_err     = zeros(3,1);
    q_err_vec = zeros(3,1);
    % w_err     = zeros(3,1);
    a_cmd     = zeros(3,1);

    %% 1) Relative position controller
    r_err = r_ref - r_rel;
    v_err = v_ref - v_rel;

    a_cmd = a_ref + Kp_pos * r_err + Kd_pos * v_err;
    F_cmd_R = m_sc * a_cmd;

    %% 2) Reference frame -> body frame
    % q : body -> reference
    % therefore F_B = C_BR' * F_R
    C_BR   = quat_to_dcm_sf(q);
    F_cmd_B = C_BR' * F_cmd_R;

    %% 3) LOS attitude controller

    % shortest path
    if q_err(1) < 0
        q_err = -q_err;
    end

    q_err_vec = q_err(2:4);

    tau_cmd_B = Kp_att * q_err_vec + Kd_att * w_err;
end


function q_out = quat_mul_sf(a, b)
% scalar-first quaternion multiplication
    q_out = [ a(1)*b(1) - a(2)*b(2) - a(3)*b(3) - a(4)*b(4);
              a(1)*b(2) + a(2)*b(1) + a(3)*b(4) - a(4)*b(3);
              a(1)*b(3) - a(2)*b(4) + a(3)*b(1) + a(4)*b(2);
              a(1)*b(4) + a(2)*b(3) - a(3)*b(2) + a(4)*b(1) ];
end


function C = quat_to_dcm_sf(q)
% scalar-first quaternion, body -> reference
    q = q / (sqrt(sum(q.^2)) + 1e-12);

    qw = q(1);
    qx = q(2);
    qy = q(3);
    qz = q(4);

    C = [1-2*(qy*qy+qz*qz),   2*(qx*qy-qw*qz),   2*(qx*qz+qw*qy);
         2*(qx*qy+qw*qz),     1-2*(qx*qx+qz*qz), 2*(qy*qz-qw*qx);
         2*(qx*qz-qw*qy),     2*(qy*qz+qw*qx),   1-2*(qx*qx+qy*qy)];
end

== matlab function model_main4/Subsystem/Subsystem1/MinOnTime_Enforcer1 ==
  settings: updateMethod=DISCRETE
  data: relay_raw input; F_gated output; t input
function F_gated = fcn(relay_raw, t)
%#codegen
% 최소 ON 시간 강제기 (MIB 기반)
% t_min_on = 0.0700 s (70 ms)
persistent t_on_start was_on;
if isempty(was_on)
    was_on     = false;
    t_on_start = 0;
end
t_min_on = 0.0700;
if relay_raw == 1 && ~was_on
    t_on_start = t;
end
if relay_raw == 1
    F_gated = 1;
elseif was_on && (t - t_on_start) < t_min_on
    F_gated = 1;   % 아직 70ms 안 됐으면 강제 ON 유지
else
    F_gated = 0;
end
was_on = (F_gated == 1);

end

== matlab function model_main4/Subsystem/Subsystem2/MinOnTime_Enforcer1 ==
  settings: updateMethod=DISCRETE
  data: relay_raw input; F_gated output; t input
function F_gated = fcn(relay_raw, t)
%#codegen
% 최소 ON 시간 강제기 (MIB 기반)
% t_min_on = 0.0700 s (70 ms)
persistent t_on_start was_on;
if isempty(was_on)
    was_on     = false;
    t_on_start = 0;
end
t_min_on = 0.0700;
if relay_raw == 1 && ~was_on
    t_on_start = t;
end
if relay_raw == 1
    F_gated = 1;
elseif was_on && (t - t_on_start) < t_min_on
    F_gated = 1;   % 아직 70ms 안 됐으면 강제 ON 유지
else
    F_gated = 0;
end
was_on = (F_gated == 1);

end

== matlab function model_main4/Subsystem/Subsystem3/MinOnTime_Enforcer1 ==
  settings: updateMethod=DISCRETE
  data: relay_raw input; F_gated output; t input
function F_gated = fcn(relay_raw, t)
%#codegen
% 최소 ON 시간 강제기 (MIB 기반)
% t_min_on = 0.0700 s (70 ms)
persistent t_on_start was_on;
if isempty(was_on)
    was_on     = false;
    t_on_start = 0;
end
t_min_on = 0.0700;
if relay_raw == 1 && ~was_on
    t_on_start = t;
end
if relay_raw == 1
    F_gated = 1;
elseif was_on && (t - t_on_start) < t_min_on
    F_gated = 1;   % 아직 70ms 안 됐으면 강제 ON 유지
else
    F_gated = 0;
end
was_on = (F_gated == 1);

end

== matlab function model_main4/Subsystem/Subsystem4/MinOnTime_Enforcer1 ==
  settings: updateMethod=DISCRETE
  data: relay_raw input; F_gated output; t input
function F_gated = fcn(relay_raw, t)
%#codegen
% 최소 ON 시간 강제기 (MIB 기반)
% t_min_on = 0.0700 s (70 ms)
persistent t_on_start was_on;
if isempty(was_on)
    was_on     = false;
    t_on_start = 0;
end
t_min_on = 0.0700;
if relay_raw == 1 && ~was_on
    t_on_start = t;
end
if relay_raw == 1
    F_gated = 1;
elseif was_on && (t - t_on_start) < t_min_on
    F_gated = 1;   % 아직 70ms 안 됐으면 강제 ON 유지
else
    F_gated = 0;
end
was_on = (F_gated == 1);

end

== matlab function model_main4/Subsystem/Subsystem5/MinOnTime_Enforcer1 ==
  settings: updateMethod=DISCRETE
  data: relay_raw input; F_gated output; t input
function F_gated = fcn(relay_raw, t)
%#codegen
% 최소 ON 시간 강제기 (MIB 기반)
% t_min_on = 0.0700 s (70 ms)
persistent t_on_start was_on;
if isempty(was_on)
    was_on     = false;
    t_on_start = 0;
end
t_min_on = 0.0700;
if relay_raw == 1 && ~was_on
    t_on_start = t;
end
if relay_raw == 1
    F_gated = 1;
elseif was_on && (t - t_on_start) < t_min_on
    F_gated = 1;   % 아직 70ms 안 됐으면 강제 ON 유지
else
    F_gated = 0;
end
was_on = (F_gated == 1);

end

== matlab function model_main4/Subsystem/Subsystem6/MinOnTime_Enforcer1 ==
  settings: updateMethod=DISCRETE
  data: relay_raw input; F_gated output; t input
function F_gated = fcn(relay_raw, t)
%#codegen
% 최소 ON 시간 강제기 (MIB 기반)
% t_min_on = 0.0700 s (70 ms)
persistent t_on_start was_on;
if isempty(was_on)
    was_on     = false;
    t_on_start = 0;
end
t_min_on = 0.0700;
if relay_raw == 1 && ~was_on
    t_on_start = t;
end
if relay_raw == 1
    F_gated = 1;
elseif was_on && (t - t_on_start) < t_min_on
    F_gated = 1;   % 아직 70ms 안 됐으면 강제 ON 유지
else
    F_gated = 0;
end
was_on = (F_gated == 1);

end

== matlab function model_main4/Subsystem/Subsystem7/MinOnTime_Enforcer1 ==
  settings: updateMethod=DISCRETE
  data: relay_raw input; F_gated output; t input
function F_gated = fcn(relay_raw, t)
%#codegen
% 최소 ON 시간 강제기 (MIB 기반)
% t_min_on = 0.0700 s (70 ms)
persistent t_on_start was_on;
if isempty(was_on)
    was_on     = false;
    t_on_start = 0;
end
t_min_on = 0.0700;
if relay_raw == 1 && ~was_on
    t_on_start = t;
end
if relay_raw == 1
    F_gated = 1;
elseif was_on && (t - t_on_start) < t_min_on
    F_gated = 1;   % 아직 70ms 안 됐으면 강제 ON 유지
else
    F_gated = 0;
end
was_on = (F_gated == 1);

end

== matlab function model_main4/Subsystem/Subsystem8/MinOnTime_Enforcer1 ==
  settings: updateMethod=DISCRETE
  data: relay_raw input; F_gated output; t input
function F_gated = fcn(relay_raw, t)
%#codegen
% 최소 ON 시간 강제기 (MIB 기반)
% t_min_on = 0.0700 s (70 ms)
persistent t_on_start was_on;
if isempty(was_on)
    was_on     = false;
    t_on_start = 0;
end
t_min_on = 0.0700;
if relay_raw == 1 && ~was_on
    t_on_start = t;
end
if relay_raw == 1
    F_gated = 1;
elseif was_on && (t - t_on_start) < t_min_on
    F_gated = 1;   % 아직 70ms 안 됐으면 강제 ON 유지
else
    F_gated = 0;
end
was_on = (F_gated == 1);

end

== matlab function model_main4/Subsystem/RCS_Relative_Position_Control_Allocation1 ==
  settings: updateMethod=DISCRETE
  data: F_cmd input; tau_cmd input; RCS_pos input; RCS_F_vec input; Tmax input; duty output; F_est output; tau_est output; F_err output; tau_err output; sat_ratio output; wF input; wT input
function [duty, F_est, tau_est, F_err, tau_err, sat_ratio] = ...
    rcs_force_torque_allocator(F_cmd, tau_cmd, RCS_pos, RCS_F_vec, Tmax, wF, wT)
%#codegen
%
% F_cmd      : [3x1] commanded force in body frame [N]
% tau_cmd    : [3x1] commanded torque in body frame [N*m]
% RCS_pos    : [3xN] thruster positions in body frame [m]
% RCS_F_vec  : [3xN] thruster direction vectors
% Tmax       : scalar, max thrust of one thruster [N]
% wF         : scalar, force tracking weight
% wT         : scalar, torque tracking weight
%
% duty       : [N x 1], 0~1
% F_est      : [3x1], achieved force [N]
% tau_est    : [3x1], achieved torque [N*m]
% F_err      : [3x1], force error [N]
% tau_err    : [3x1], torque error [N*m]
% sat_ratio  : saturated thruster ratio

    N = size(RCS_pos, 2);

    duty      = zeros(N,1);
    F_est     = zeros(3,1);
    tau_est   = zeros(3,1);
    F_err     = zeros(3,1);
    tau_err   = zeros(3,1);
    sat_ratio = 0;

    Fmat = zeros(3, N);
    Tmat = zeros(3, N);

    for i = 1:N
        dir_i = RCS_F_vec(:,i);
        nrm   = sqrt(sum(dir_i.^2));

        if nrm > 1e-12
            dir_i = dir_i / nrm;
        else
            dir_i = [0;0;0];
        end

        Fi = Tmax * dir_i;
        Ti = cross3(RCS_pos(:,i), Fi);

        Fmat(:,i) = Fi;
        Tmat(:,i) = Ti;
    end

    % Solve:
    % min || wF*(Fmat*u - F_cmd) ||^2 + || wT*(Tmat*u - tau_cmd) ||^2
    % s.t. 0 <= u <= 1

    A = [wF * Fmat;
         wT * Tmat];

    b = [wF * F_cmd;
         wT * tau_cmd];

    H = A' * A + 1e-8 * eye(N);
    g = A' * b;

    alpha = 1.0 / (trace(H) + 1e-9);
    u = zeros(N,1);

    for k = 1:150
        grad = H * u - g;
        u    = u - alpha * grad;

        for j = 1:N
            if u(j) < 0
                u(j) = 0;
            elseif u(j) > 1
                u(j) = 1;
            end
        end
    end

    duty    = u;
    F_est   = Fmat * duty;
    tau_est = Tmat * duty;

    F_err   = F_cmd   - F_est;
    tau_err = tau_cmd - tau_est;

    sat_ratio = sum(duty > 0.999) / N;
end


function c = cross3(a, b)
    c = [ a(2)*b(3) - a(3)*b(2);
          a(3)*b(1) - a(1)*b(3);
          a(1)*b(2) - a(2)*b(1) ];
end

== matlab function model_main4/SS Attitude Control wrt ECI ==
  settings: updateMethod=DISCRETE
  data: q_err input; RW_cmd output; w_err input; As input; Kp_rw input; Kd_rw input; Ki_rw input
function RW_cmd  = Att_PD_Control(q_err, w_err, As,Kp_rw,Kd_rw,Ki_rw)

persistent I_save
persistent flg

if isempty(flg)
    flg = 1;
    I_save = [0 0 0]';
end
 
% K3 = 0.025*diag([1 1 1]);

q_e_v = [q_err(2), q_err(3), q_err(4)]';

u = Kp_rw*q_e_v + Kd_rw*w_err + Ki_rw*I_save;

% RW_cmd = pinv(As)*-u;
RW_cmd = u; 

I_save = I_save + (q_e_v*0.01);

end
